simulink model "PIDQuadControl"  (R2014b)
settings: Solver=ode45  StartTime=0.0  StopTime=20  RelTol=1e-3
values from neighbouring files (symbols this model uses):
  b = 3.13e-5    (= 3.13e-05)    [Parrametresnnlineaire.m]
  d = 7.50e-7    (= 7.5e-07)    [Parrametresnnlineaire.m]
  g = 9.81    [Parrametresnnlineaire.m]
  Ix = 0.0075    [Parrametresnnlineaire.m]
  Iy = 0.0075    [Parrametresnnlineaire.m]
  Iz = 0.013    [Parrametresnnlineaire.m]
  Jr = 6e-5    (= 6e-05)    [Parrametresnnlineaire.m]
  l = 0.23    [Parrametresnnlineaire.m]
  m = 0.65    [Parrametresnnlineaire.m]
settings Model: Creator=Khadija  LastModifiedBy=Khadija
settings SolverCC: ZeroCrossAlgorithm=Adaptive

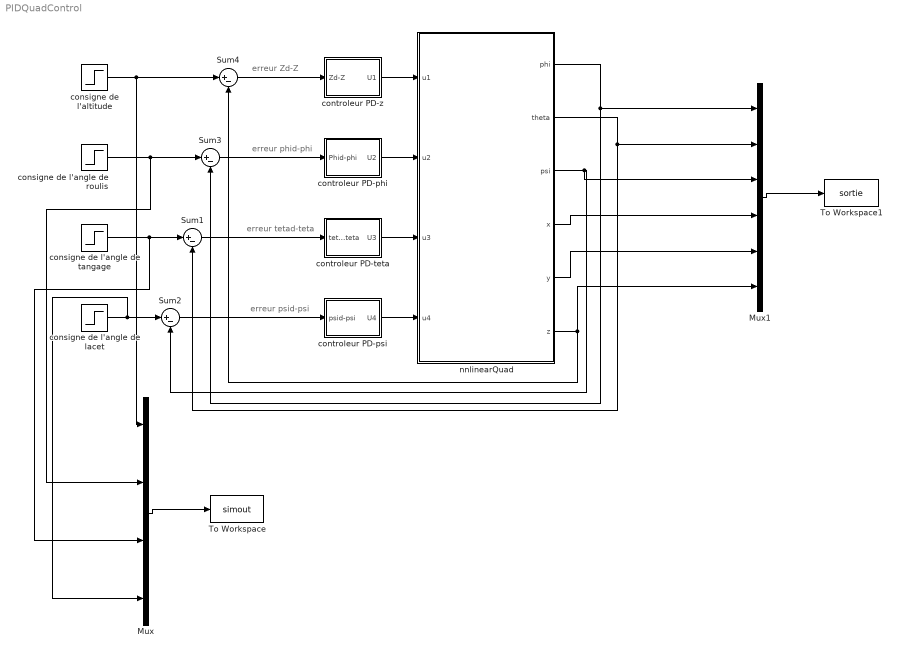
== system PIDQuadControl ==
  note: erreur psid-psi
  note: erreur tetad-teta
  note: erreur Zd-Z
  note: erreur phid-phi
  Mux : Mux
  Mux1 : Mux  Inputs=6
  Sum{1..4} (4 alike) : Sum  Inputs=|+-
  To Workspace : ToWorkspace  VariableName=simout  SaveFormat=Structure With Time  SampleTime=-1
  To Workspace1 : ToWorkspace  VariableName=sortie  SaveFormat=Structure With Time  SampleTime=-1
  consigne de l'altitude : Step  SampleTime=0
  consigne de l'angle de lacet : Step  After=0.5  SampleTime=0
  consigne de l'angle de roulis : Step  After=0.5  SampleTime=0
  consigne de l'angle de tangage : Step  After=0.5  SampleTime=0
  controleur PD-phi : Subsystem
  controleur PD-psi : Subsystem
  controleur PD-teta : Subsystem
  "controleur PD-z " : Subsystem
  nnlinearQuad : Subsystem
  wires:
  nnlinearQuad/6(z) -> Sum4/2, Mux1/6
  nnlinearQuad/3(psi) -> Mux1/3, Sum2/2
  nnlinearQuad/1("phi ") -> Mux1/1, Sum3/2
  nnlinearQuad/2(theta) -> Mux1/2, Sum1/2
  Sum3/1 -> controleur PD-phi/1(Phid-phi)
  consigne de l'angle de roulis/1 -> Mux/2, Sum3/1
  "controleur PD-z "/1(U1) -> nnlinearQuad/1(u1)
  controleur PD-phi/1(U2) -> nnlinearQuad/2(u2)
  controleur PD-teta/1("U3 ") -> nnlinearQuad/3(u3)
  controleur PD-psi/1(U4) -> nnlinearQuad/4(u4)
  consigne de l'angle de tangage/1 -> Mux/3, Sum1/1
  Sum2/1 -> controleur PD-psi/1(psid-psi)
  Sum1/1 -> controleur PD-teta/1(tetad-teta)
  Sum4/1 -> "controleur PD-z "/1(Zd-Z)
  consigne de l'angle de lacet/1 -> Mux/4, Sum2/1
  consigne de l'altitude/1 -> Sum4/1, Mux/1
  Mux/1 -> To Workspace/1
  Mux1/1 -> To Workspace1/1
  nnlinearQuad/4(x) -> Mux1/4
  nnlinearQuad/5(y) -> Mux1/5

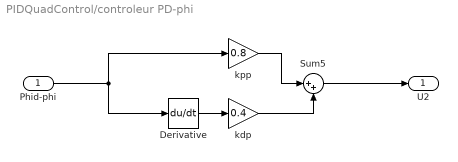
== system PIDQuadControl/controleur PD-phi ==
  Phid-phi : Inport
  Derivative : Derivative
  Sum5 : Sum  Inputs=|++
  kdp : Gain  Gain=0.4
  kpp : Gain  Gain=0.8
  U2 : Outport
  wires:
  Derivative/1 -> kdp/1
  Phid-phi/1 -> Derivative/1, kpp/1
  kdp/1 -> Sum5/2
  Sum5/1 -> U2/1
  kpp/1 -> Sum5/1

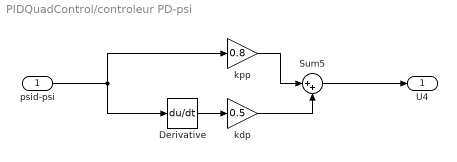
== system PIDQuadControl/controleur PD-psi ==
  psid-psi : Inport
  Derivative : Derivative
  Sum5 : Sum  Inputs=|++
  kdp : Gain  Gain=0.5
  kpp : Gain  Gain=0.8
  U4 : Outport
  wires:
  Derivative/1 -> kdp/1
  psid-psi/1 -> Derivative/1, kpp/1
  kdp/1 -> Sum5/2
  Sum5/1 -> U4/1
  kpp/1 -> Sum5/1

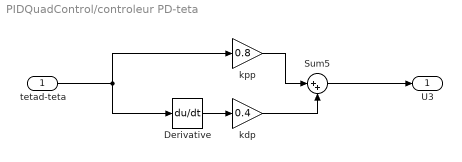
== system PIDQuadControl/controleur PD-teta ==
  tetad-teta : Inport
  Derivative : Derivative
  Sum5 : Sum  Inputs=|++
  kdp : Gain  Gain=0.4
  kpp : Gain  Gain=0.8
  "U3 " : Outport
  wires:
  kpp/1 -> Sum5/1
  Sum5/1 -> "U3 "/1
  kdp/1 -> Sum5/2
  tetad-teta/1 -> kpp/1, Derivative/1
  Derivative/1 -> kdp/1

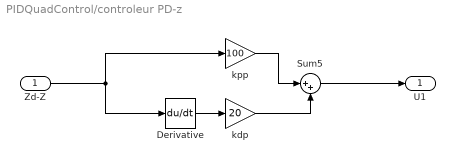
== system PIDQuadControl/controleur PD-z  ==
  Zd-Z : Inport
  Derivative : Derivative
  Sum5 : Sum  Inputs=|++
  kdp : Gain  Gain=20
  kpp : Gain  Gain=100
  U1 : Outport
  wires:
  kpp/1 -> Sum5/1
  Sum5/1 -> U1/1
  kdp/1 -> Sum5/2
  Zd-Z/1 -> kpp/1, Derivative/1
  Derivative/1 -> kdp/1

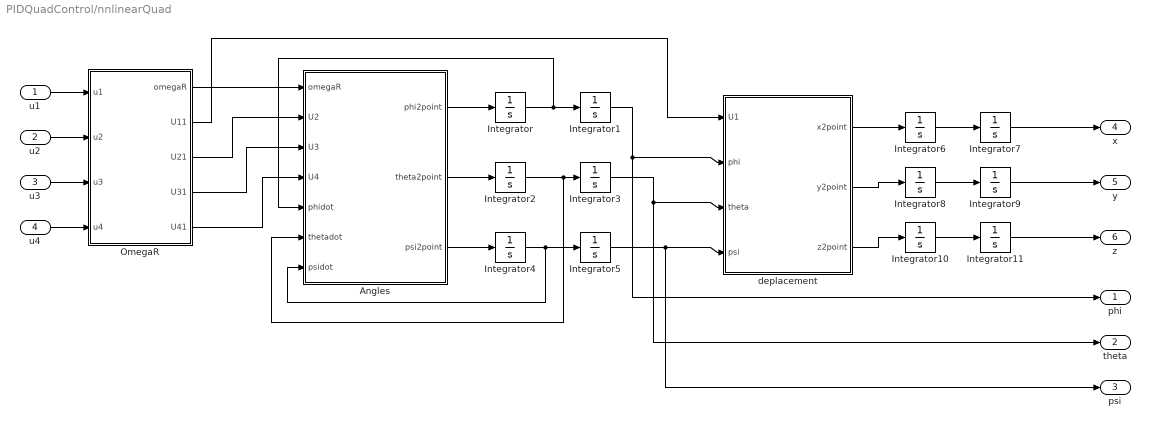
== system PIDQuadControl/nnlinearQuad ==
  u1 : Inport
  u2 : Inport  Port=2
  u3 : Inport  Port=3
  u4 : Inport  Port=4
  Angles : Subsystem
  Integrator : Integrator  UpperSaturationLimit=0.5  LowerSaturationLimit=-0.5
  Integrator{1,3,5,7,9,11} (6 alike) : Integrator
  Integrator10 : Integrator  UpperSaturationLimit=1  LowerSaturationLimit=-1
  Integrator2 : Integrator  UpperSaturationLimit=0.5  LowerSaturationLimit=-0.5
  Integrator4 : Integrator  UpperSaturationLimit=0.5  LowerSaturationLimit=-0.5
  Integrator6 : Integrator  UpperSaturationLimit=1  LowerSaturationLimit=-1
  Integrator8 : Integrator  UpperSaturationLimit=1  LowerSaturationLimit=-1
  OmegaR : Subsystem
  deplacement : Subsystem
  "phi " : Outport
  theta : Outport  Port=2
  psi : Outport  Port=3
  x : Outport  Port=4
  y : Outport  Port=5
  z : Outport  Port=6
  wires:
  u1/1 -> OmegaR/1(u1)
  u4/1 -> OmegaR/4(u4)
  u2/1 -> OmegaR/2(u2)
  u3/1 -> OmegaR/3(u3)
  Integrator10/1 -> Integrator11/1
  Integrator8/1 -> Integrator9/1
  Integrator6/1 -> Integrator7/1
  Integrator7/1 -> x/1
  OmegaR/2("U11 ") -> deplacement/1(U1)
  deplacement/3(z2point) -> Integrator10/1
  deplacement/1(x2point) -> Integrator6/1
  Integrator9/1 -> y/1
  deplacement/2(y2point) -> Integrator8/1
  Integrator2/1 -> Angles/6(thetadot), Integrator3/1
  Integrator4/1 -> Angles/7(psidot), Integrator5/1
  Integrator3/1 -> deplacement/3(theta), theta/1
  Angles/2(theta2point) -> Integrator2/1
  Angles/3(psi2point) -> Integrator4/1
  Angles/1("phi2point ") -> Integrator/1
  Integrator/1 -> Angles/5(phidot), Integrator1/1
  Integrator1/1 -> "phi "/1, deplacement/2(phi)
  OmegaR/4(U31) -> Angles/3(U3)
  OmegaR/1(omegaR) -> Angles/1(omegaR)
  OmegaR/3(U21) -> Angles/2(U2)
  OmegaR/5(U41) -> Angles/4("U4 ")
  Integrator11/1 -> z/1
  Integrator5/1 -> psi/1, deplacement/4(psi)

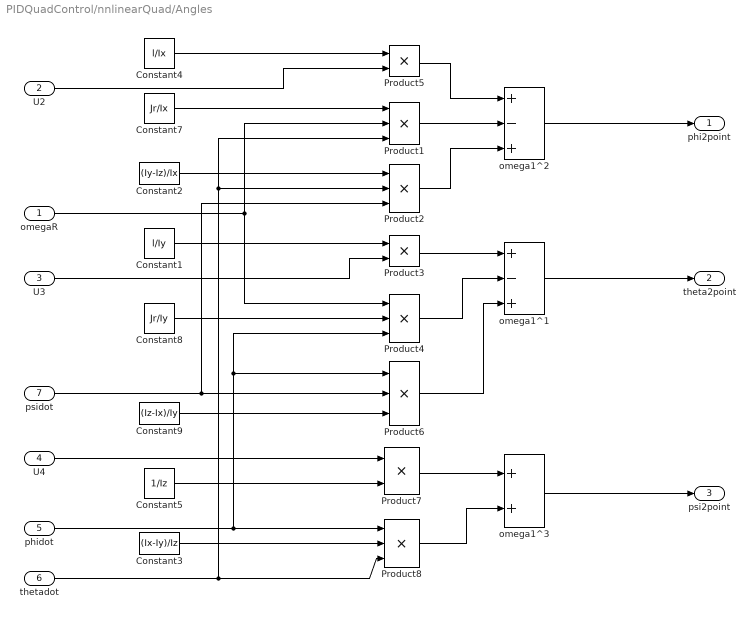
== system PIDQuadControl/nnlinearQuad/Angles ==
  omegaR : Inport
  U2 : Inport  Port=2
  U3 : Inport  Port=3
  "U4 " : Inport  Port=4
  phidot : Inport  Port=5
  thetadot : Inport  Port=6
  psidot : Inport  Port=7
  Constant1 : Constant  Value=l/Iy
  Constant2 : Constant  Value=(Iy-Iz)/Ix
  Constant3 : Constant  Value=(Ix-Iy)/Iz
  Constant4 : Constant  Value=l/Ix
  Constant5 : Constant  Value=1/Iz
  Constant7 : Constant  Value=Jr/Ix
  Constant8 : Constant  Value=Jr/Iy
  Constant9 : Constant  Value=(Iz-Ix)/Iy
  Product{1..2,4,6,8} (5 alike) : Product  Inputs=***
  Product3 : Product  Inputs=**
  Product5 : Product  Inputs=**
  Product7 : Product  Inputs=**
  omega1^1 : Sum  Inputs=+-+
  omega1^2 : Sum  Inputs=+-+
  omega1^3 : Sum
  "phi2point " : Outport
  theta2point : Outport  Port=2
  psi2point : Outport  Port=3
  wires:
  Constant2/1 -> Product2/1
  Constant4/1 -> Product5/1
  Constant7/1 -> Product1/1
  omegaR/1 -> Product4/1, Product1/2
  U2/1 -> Product5/2
  U3/1 -> Product3/2
  Constant9/1 -> Product6/3
  psidot/1 -> Product2/3, Product6/2
  thetadot/1 -> Product1/3, Product2/2, Product8/3
  phidot/1 -> Product4/3, Product6/1, Product8/1
  Product1/1 -> omega1^2/2
  Constant1/1 -> Product3/1
  Product7/1 -> omega1^3/1
  Product3/1 -> omega1^1/1
  Constant8/1 -> Product4/2
  Product6/1 -> omega1^1/3
  Product5/1 -> omega1^2/1
  Product2/1 -> omega1^2/3
  Product4/1 -> omega1^1/2
  omega1^2/1 -> "phi2point "/1
  omega1^1/1 -> theta2point/1
  omega1^3/1 -> psi2point/1
  Constant5/1 -> Product7/2
  "U4 "/1 -> Product7/1
  Product8/1 -> omega1^3/2
  Constant3/1 -> Product8/2

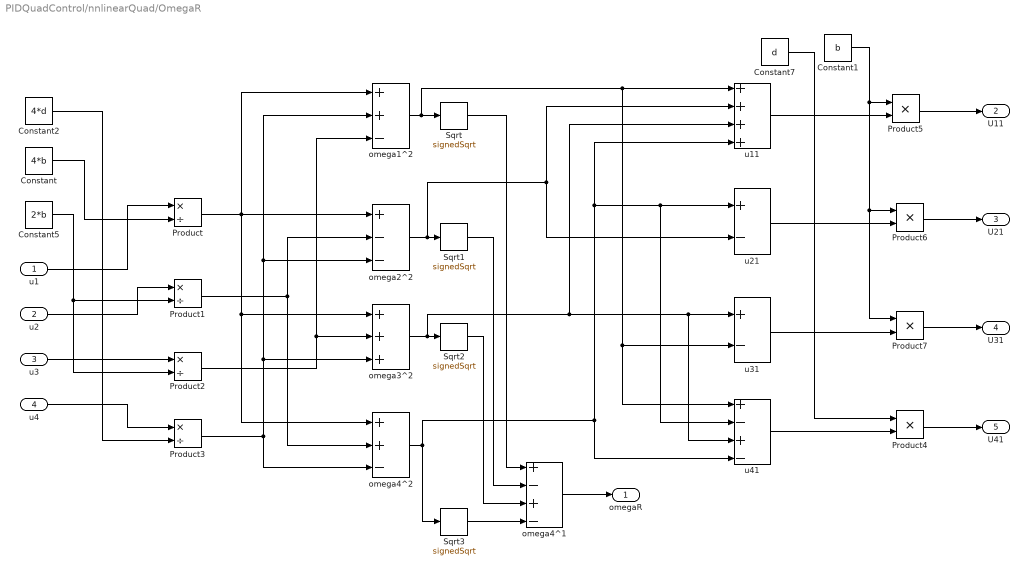
== system PIDQuadControl/nnlinearQuad/OmegaR ==
  u1 : Inport
  u2 : Inport  Port=2
  u3 : Inport  Port=3
  u4 : Inport  Port=4
  Constant : Constant  Value=4*b
  Constant1 : Constant  Value=b
  Constant2 : Constant  Value=4*d
  Constant5 : Constant  Value=2*b
  Constant7 : Constant  Value=d
  Product{,1..3} (4 alike) : Product  Inputs=*/
  Product{4..7} (4 alike) : Product  Inputs=**
  Sqrt{,1..3} (4 alike) : Sqrt  Operator=signedSqrt  OutputSignalType=real  SaturateOnIntegerOverflow=on
  omega1^2 : Sum  Inputs=++-
  omega2^2 : Sum  Inputs=+--
  omega3^2 : Sum  Inputs=+++
  omega4^1 : Sum  Inputs=+-+-
  omega4^2 : Sum  Inputs=++-
  u11 : Sum  Inputs=++++
  u21 : Sum  Inputs=+-
  u31 : Sum  Inputs=+-
  "u41 " : Sum  Inputs=+-+-
  omegaR : Outport
  "U11 " : Outport  Port=2
  U21 : Outport  Port=3
  U31 : Outport  Port=4
  U41 : Outport  Port=5
  wires:
  u11/1 -> Product5/2
  Product5/1 -> "U11 "/1
  Product7/1 -> U31/1
  omega4^2/1 -> u21/1, "u41 "/2, u11/4, "u41 "/4, Sqrt3/1
  Product1/1 -> omega4^2/2, omega2^2/2
  Product6/1 -> U21/1
  omega2^2/1 -> u11/2, u21/2, Sqrt1/1
  Sqrt3/1 -> omega4^1/4
  Product2/1 -> omega1^2/3, omega3^2/2
  Constant5/1 -> Product2/2, Product1/2
  omega1^2/1 -> u11/1, u31/2, "u41 "/1, Sqrt/1
  Sqrt1/1 -> omega4^1/2
  Product4/1 -> U41/1
  u31/1 -> Product7/2
  u21/1 -> Product6/2
  Constant/1 -> Product/2
  u3/1 -> Product2/1
  Product3/1 -> omega4^2/3, omega3^2/3, omega2^2/3, omega1^2/2
  u4/1 -> Product3/1
  Constant1/1 -> Product7/1, Product6/1, Product5/1
  "u41 "/1 -> Product4/2
  u1/1 -> Product/1
  Sqrt2/1 -> omega4^1/3
  Constant2/1 -> Product3/2
  Constant7/1 -> Product4/1
  Product/1 -> omega4^2/1, omega3^2/1, omega2^2/1, omega1^2/1
  u2/1 -> Product1/1
  omega3^2/1 -> u11/3, "u41 "/3, u31/1, Sqrt2/1
  Sqrt/1 -> omega4^1/1
  omega4^1/1 -> omegaR/1

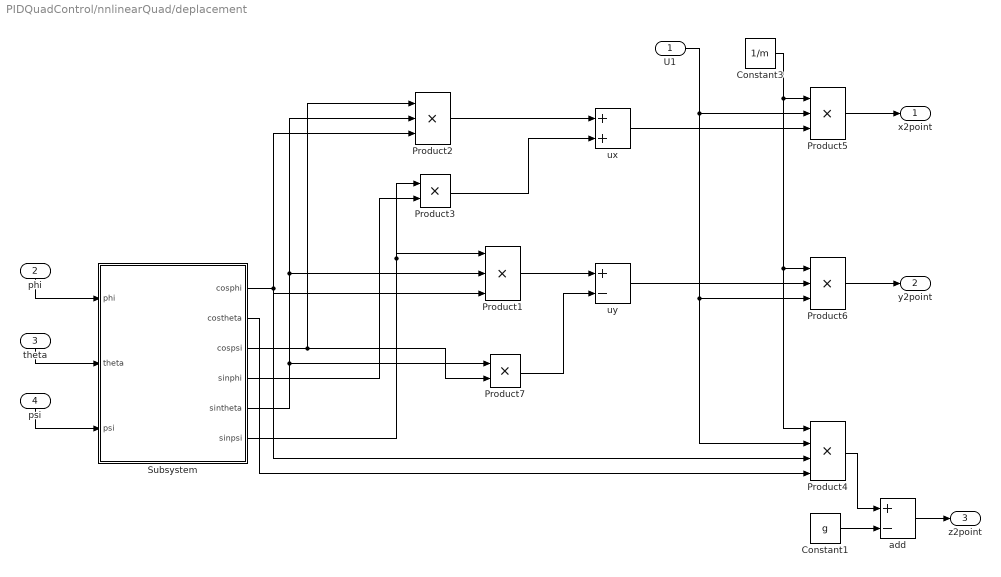
== system PIDQuadControl/nnlinearQuad/deplacement ==
  U1 : Inport
  phi : Inport  Port=2
  theta : Inport  Port=3
  psi : Inport  Port=4
  Constant1 : Constant  Value=g
  Constant3 : Constant  Value=1/m
  Product{1..2,5..6} (4 alike) : Product  Inputs=***
  Product3 : Product  Inputs=**
  Product4 : Product  Inputs=****
  Product7 : Product  Inputs=**
  Subsystem : Subsystem
  add : Sum  Inputs=+-
  ux : Sum
  uy : Sum  Inputs=+-
  x2point : Outport
  y2point : Outport  Port=2
  z2point : Outport  Port=3
  wires:
  Product4/1 -> add/1
  ux/1 -> Product5/3
  Product6/1 -> y2point/1
  uy/1 -> Product6/2
  U1/1 -> Product5/2, Product6/3, Product4/2
  add/1 -> z2point/1
  Constant3/1 -> Product5/1, Product4/1, Product6/1
  Product5/1 -> x2point/1
  Constant1/1 -> add/2
  phi/1 -> Subsystem/1(phi)
  theta/1 -> Subsystem/2(theta)
  psi/1 -> Subsystem/3(psi)
  Product2/1 -> ux/1
  Product3/1 -> ux/2
  Subsystem/3(cospsi) -> Product2/1, Product7/2
  Subsystem/5(sintheta) -> Product7/1, Product2/2, Product1/2
  Subsystem/6(sinpsi) -> Product3/1, Product1/1
  Subsystem/4(sinphi) -> Product3/2
  Product1/1 -> uy/1
  Product7/1 -> uy/2
  Subsystem/1(cosphi) -> Product4/3, Product2/3, Product1/3
  Subsystem/2(costheta) -> Product4/4

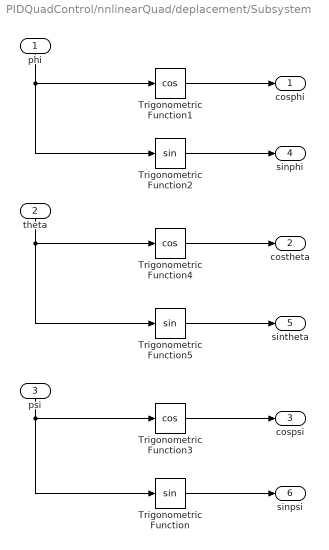
== system PIDQuadControl/nnlinearQuad/deplacement/Subsystem ==
  phi : Inport
  theta : Inport  Port=2
  psi : Inport  Port=3
  Trigonometric Function : Trigonometry
  Trigonometric Function1 : Trigonometry  Operator=cos
  Trigonometric Function2 : Trigonometry
  Trigonometric Function3 : Trigonometry  Operator=cos
  Trigonometric Function4 : Trigonometry  Operator=cos
  Trigonometric Function5 : Trigonometry
  cosphi : Outport
  costheta : Outport  Port=2
  cospsi : Outport  Port=3
  sinphi : Outport  Port=4
  sintheta : Outport  Port=5
  sinpsi : Outport  Port=6
  wires:
  Trigonometric Function2/1 -> sinphi/1
  psi/1 -> Trigonometric Function3/1, Trigonometric Function/1
  phi/1 -> Trigonometric Function2/1, Trigonometric Function1/1
  theta/1 -> Trigonometric Function5/1, Trigonometric Function4/1
  Trigonometric Function5/1 -> sintheta/1
  Trigonometric Function/1 -> sinpsi/1
  Trigonometric Function3/1 -> cospsi/1
  Trigonometric Function1/1 -> cosphi/1
  Trigonometric Function4/1 -> costheta/1
